simulink model "ganil_hot_part"  (R2016b)
settings: Solver=VariableStepAuto  StartTime=0.0  StopTime=1e6  RelTol=1e-3  EnableMultiTasking=on
libraries: simCryogenics_lib x21, nesl_utility x19
settings Model: Creator=FB229602  LastModifiedBy=trinhvv-admin
settings OptimizationCC: LifeSpan=inf
settings DebuggingCC: SFUnexpectedBacktrackingDiag=warning  SFNoUnconditionalDefaultTransitionDiag=warning  SFExecutionAtInitializationDiag=none
settings GRTTargetCC: TargetLangStandard=C89/C90 (ANSI)  GeneratePreprocessorConditionals=Disable all
settings ConfigComp: CovMetricSettings=dw  CovHtmlReporting=on  CovSaveCumulativeToWorkspaceVar=on  CovSaveSingleToWorkspaceVar=on  CovExternalEMLEnable=off
settings SimscapeCC: SimscapeLogType=all

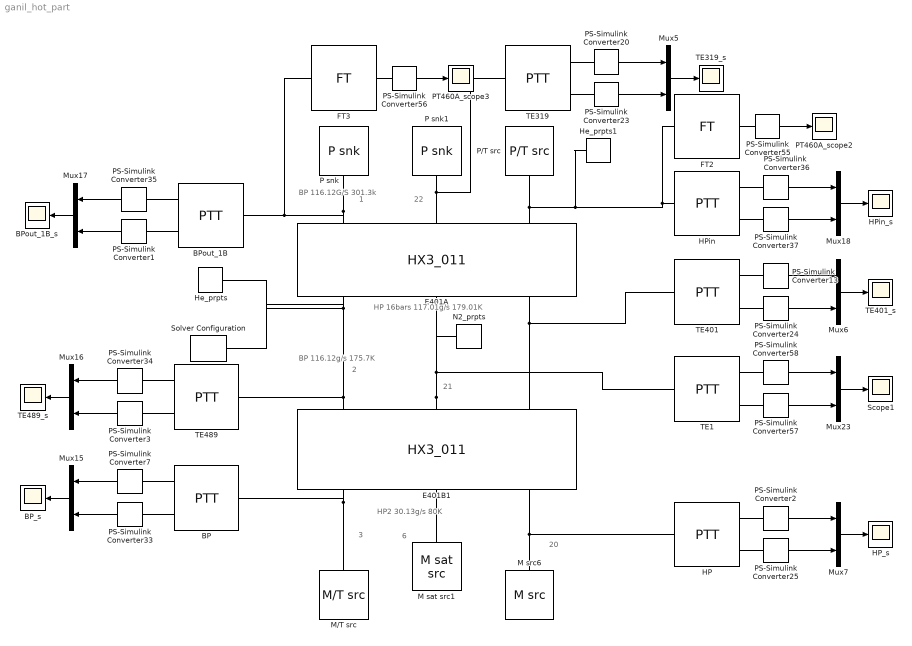
== system ganil_hot_part ==
  note: 6
  note: 20
  note: 21
  note: 22
  note: 3
  note: 2
  note: 1
  note: BP
      | 116.12G/S
      | 301.3k
  note: HP
      | 16bars
      | 117.01g/s
      | 179.01K
  note: BP
      | 116.12g/s
      | 175.7K
  note: HP2
      | 30.13g/s
      | 80K
  BP : simCryogenics_lib/Sensors/PTT
  BP_s : Scope
  BPout_1B : simCryogenics_lib/Sensors/PTT
  BPout_1B_s : Scope
  E401A : simCryogenics_lib/Elements/HX3_011  N=9  Vh=0.118 m^3  Vm=0.055 m^3  Vc=0.008 km^3  M=281 kg  Kh=0.062/0.11612 s*bar/kg  Km=0.033/0.11701 s*bar/kg  Kc=0.021/.0026 s*bar/kg  hh_m=0 J/s/K  hh_c=2.5e4 J/s/K  hm_c=250 J/s/K  Th0=300 K  Ph0=15 bar  Mh0=0.11612 kg/s  Tm0=175 K  Pm0=1 bar  Mm0=0.0026 kg/s  Tc0=175.7 K  Pc0=1.05 bar  Mc0=0.11612 kg/s  sensh=0  sensm=1  sensc=1
  E401B1 : simCryogenics_lib/Elements/HX3_011  N=9  Vh=0.133 m^3  Vm=0.062 m^3  Vc=0.012 m^3  M=195 kg  Kh=0.0255/0.11612 s*bar/kg  Km=0.014/0.11701 s*bar/kg  Kc=0.002/0.0026 s*bar/kg  hh_m=5000 J/s/K  hh_c=3e4 J/s/K  hm_c=1 J/s/K  Th0=179 K  Ph0=14.4 bar  Mh0=0.116 kg/s  Tm0=79 K  Pm0=1.1 bar  Mm0=0.0026 kg/s  Tc0=79.2 K  Pc0=1.05 bar  Mc0=0.116 kg/s  sensh=0  sensm=1  sensc=1
  FT2 : simCryogenics_lib/Sensors/FT
  FT3 : simCryogenics_lib/Sensors/FT
  HP : simCryogenics_lib/Sensors/PTT
  HP_s : Scope
  HPin : simCryogenics_lib/Sensors/PTT
  HPin_s : Scope
  He_prpts : simCryogenics_lib/Utilities/He_prpts  P_min=0.1 bar  P_max=30 bar  T_min=3 K  T_max=320 K  N=100  Mol=4.0026 * 10 ^ (- 3) kg/mol
  He_prpts1 : simCryogenics_lib/Utilities/He_prpts  P_min=0.1 bar  P_max=30 bar  T_min=3 K  T_max=320 K  N=100  Mol=4.0026 * 10 ^ (- 3) kg/mol
  M sat src1 : simCryogenics_lib/Sources_Sinks/M sat src  M=0.007 kg/s  Xmix=0
  M src6 : simCryogenics_lib/Sources_Sinks/M src  M=0.116 kg/s
  M/T src : simCryogenics_lib/Sources_Sinks/M//T src  M=0.116 kg/s  T=78 K
  Mux{5..7,15..18,23} (8 alike) : Mux  Inputs=2
  N2_prpts : simCryogenics_lib/Utilities/N2_prpts  P_min=0.5 bar  T_min=70 K  T_max=320 K  P_max=20 bar  Mol=4.0026 * (10 ^ (- 3)) kg/mol
  P snk : simCryogenics_lib/Sources_Sinks/P snk  P=1.05 bar
  P snk1 : simCryogenics_lib/Sources_Sinks/P snk  P=1.05 bar
  P/T src : simCryogenics_lib/Sources_Sinks/P//T src  P=14.73 bar  T=305 K
  PS-Simulink Converter{1..3,7,13,20,23..25,33..37,55..58} (18 alike) : nesl_utility/PS-Simulink Converter  PhysicalDomain=network_engine_domain  SubClassName=ps_output  LeftPortType=input  RightPortType=output  PseudoPeriodic=off  Frequencies=[]  Unit=1  AffineConversion=off
  PT460A_scope2 : Scope
  PT460A_scope3 : Scope
  Scope1 : Scope
  Solver Configuration : nesl_utility/Solver Configuration  PhysicalDomain=network_engine_domain  SubClassName=solver  LeftPortType=input  RightPortType=generic  Accelerate=off  Tones=[]  Harmonics=[]  SimulateNoise=off  Profile=off  UseLocalSampling=off  EnableSwitchedLinearOptims=on  FrequencyDomain=off  UseCCode=off  RelTol=0.001  AbsTol=1e-06  MinStep=1e-09  ToWorkspace=off  RevertToSquareIcSolve=off  NumHomotopyIterations=100  PhasorMode=off  PhasorModeNumHarmonics=1  OverrideAbsTol=off  DoDC=off  ResidualTolerance=1e-09  UseLocalSolver=off  LocalSolverChoice=NE_BACKWARD_EULER_ADVANCER  LocalSolverSampleTime=0.001  DoFixedCost=off  MaxNonlinIter=3  MaxModeIter=2  LinearAlgebra=Sparse  DelaysMemoryBudget=1024  AutomaticFiltering=on  FilteringTimeConstant=0.001
  TE{1,319,401,489} (4 alike) : simCryogenics_lib/Sensors/PTT
  TE319_s : Scope
  TE401_s : Scope
  TE489_s : Scope
  wires:
  PS-Simulink Converter20/1 -> Mux5/1
  PS-Simulink Converter23/1 -> Mux5/2
  Mux5/1 -> TE319_s/1
  PS-Simulink Converter13/1 -> Mux6/1
  PS-Simulink Converter24/1 -> Mux6/2
  Mux6/1 -> TE401_s/1
  PS-Simulink Converter25/1 -> Mux7/2
  Mux7/1 -> HP_s/1
  PS-Simulink Converter2/1 -> Mux7/1
  Mux15/1 -> BP_s/1
  PS-Simulink Converter7/1 -> Mux15/1
  PS-Simulink Converter33/1 -> Mux15/2
  Mux16/1 -> TE489_s/1
  PS-Simulink Converter34/1 -> Mux16/1
  PS-Simulink Converter3/1 -> Mux16/2
  Mux17/1 -> BPout_1B_s/1
  PS-Simulink Converter35/1 -> Mux17/1
  PS-Simulink Converter1/1 -> Mux17/2
  PS-Simulink Converter36/1 -> Mux18/1
  PS-Simulink Converter37/1 -> Mux18/2
  Mux18/1 -> HPin_s/1
  PS-Simulink Converter55/1 -> PT460A_scope2/1
  PS-Simulink Converter56/1 -> PT460A_scope3/1
  PS-Simulink Converter57/1 -> Mux23/2
  Mux23/1 -> Scope1/1
  PS-Simulink Converter58/1 -> Mux23/1
  connections:
  BPout_1B/LConn1 -- P snk/RConn1 -- E401A/LConn1 -- FT3/LConn1
  BP/LConn1 -- E401B1/RConn1 -- M/T src/RConn1
  E401B1/LConn1 -- TE489/LConn1 -- He_prpts/RConn1 -- Solver Configuration/RConn1 -- E401A/RConn1
  M src6/RConn1 -- HP/LConn1 -- E401B1/RConn3
  FT2/LConn1 -- HPin/LConn1 -- He_prpts1/RConn1 -- P/T src/RConn1 -- E401A/LConn3
  TE401/LConn1 -- E401A/RConn3 -- E401B1/LConn3
  M sat src1/RConn1 -- E401B1/RConn2
  TE319/LConn1 -- P snk1/RConn1 -- E401A/LConn2
  E401B1/LConn2 -- TE1/LConn1 -- E401A/RConn2 -- N2_prpts/RConn1
  PS-Simulink Converter55/LConn1 -- FT2/RConn1
  PS-Simulink Converter20/LConn1 -- TE319/RConn1
  HP/RConn1 -- PS-Simulink Converter2/LConn1
  BP/RConn2 -- PS-Simulink Converter33/LConn1
  PS-Simulink Converter24/LConn1 -- TE401/RConn2
  PS-Simulink Converter37/LConn1 -- HPin/RConn2
  PS-Simulink Converter13/LConn1 -- TE401/RConn1
  PS-Simulink Converter57/LConn1 -- TE1/RConn2
  PS-Simulink Converter25/LConn1 -- HP/RConn2
  BPout_1B/RConn2 -- PS-Simulink Converter1/LConn1
  TE489/RConn2 -- PS-Simulink Converter3/LConn1
  PS-Simulink Converter7/LConn1 -- BP/RConn1
  PS-Simulink Converter35/LConn1 -- BPout_1B/RConn1
  PS-Simulink Converter58/LConn1 -- TE1/RConn1
  PS-Simulink Converter56/LConn1 -- FT3/RConn1
  PS-Simulink Converter23/LConn1 -- TE319/RConn2
  PS-Simulink Converter34/LConn1 -- TE489/RConn1
  PS-Simulink Converter36/LConn1 -- HPin/RConn1
